simulink model "Final"  (R2022a)
settings: Solver=FixedStepAuto  StartTime=0.0  StopTime=10.0  FixedStep=1e-3  RelTol=1e-3  EnableMultiTasking=on
undefined symbols (not defined in the file): D0, D1, D10, D11, D12, D13, D2, D3, D4, D5, D6, D7, D8, D9, PTA0, PTA1, PTA2, PTB23, PTB9, PTC16, PTC17, PTC2, PTC3, PTC4, PTD0, PTD1, PTD2, PTD3
libraries: frdmk64flib x15
settings Model: ExtModeTrigDuration=5  Creator=pauls  LastModifiedBy=pauls
settings OptimizationCC: EnhancedBackFolding=on  PassReuseOutputArgsAs=Individual arguments  ZeroExternalMemoryAtStartup=off  ZeroInternalMemoryAtStartup=off  MaxStackSize=64  OptimizeBlockOrder=speed  DifferentSizesBufferReuse=on  OptimizationCustomize=off  EfficientTunableParamExpr=on
settings DebuggingCC: ParameterTunabilityLossMsg=error
settings HardwareCC: ProdBitPerPointer=32  ProdBitPerSizeT=32  ProdBitPerPtrDiffT=32  ProdLargestAtomicInteger=Long  ProdLargestAtomicFloat=Double  ProdWordSize=32  ProdHWDeviceType=ARM Compatible->ARM Cortex
settings SFSimCC: MATLABDynamicMemAlloc=off
settings RTWCC: SystemTargetFile=ert.tlc  HardwareBoard=NXP FRDM-K64F  TLCOptions="-aInlineSetEventsForThisBaseRateFcn=TLC_FALSE -aSuppressMultiTaskScheduler=TLC_FALSE  -aRateBasedStepFcn=0"  TemplateMakefile=ert_default_tmf  Toolchain=GNU Tools for ARM Embedded Processors
settings CodeAppCC: ForceParamTrailComments=on  IgnoreCustomStorageClasses=off  OperatorAnnotations=on  SimulinkDataObjDesc=on  SFDataObjDesc=on  InsertBlockDesc=on
settings ERTTargetCC: ExtModeTransport=4  ExtModeMexFile=sendToCommService

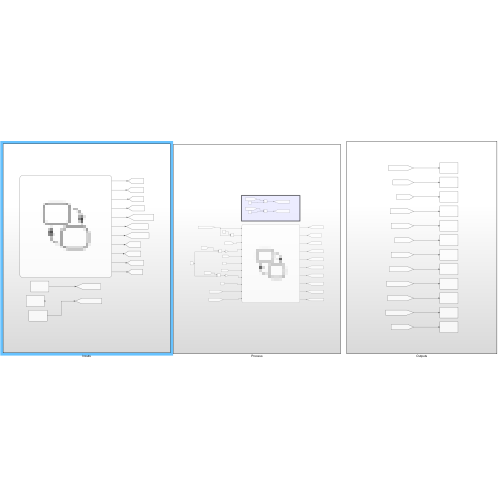
[thumbnail: Simulink's stored preview of the top-level diagram]
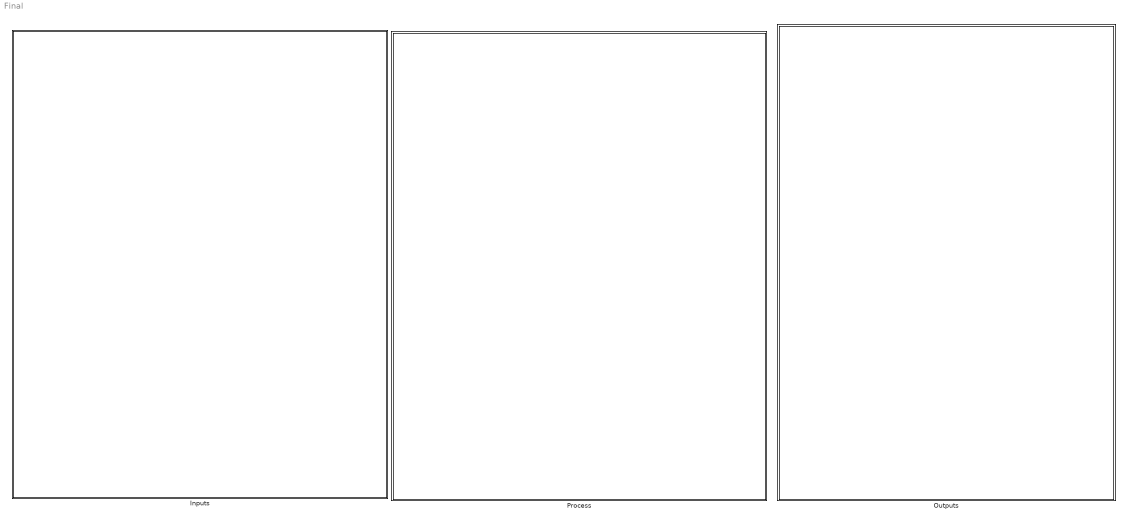
== system Final ==
  Inputs : Subsystem
  Outputs : Subsystem
  Process : Subsystem

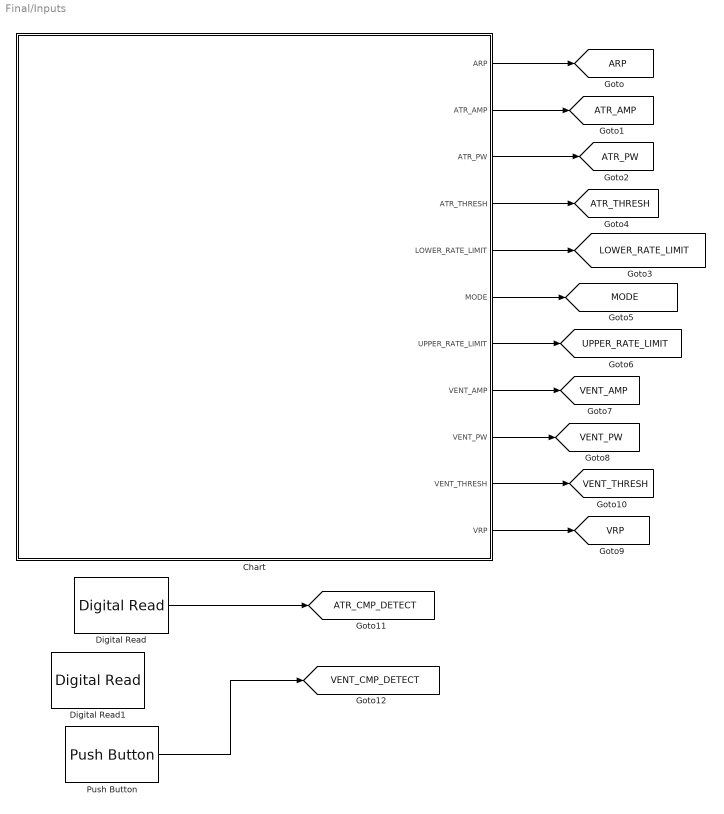
== system Final/Inputs ==
  Chart : Stateflow chart  TreatAsAtomicUnit=on
  Digital Read : frdmk64flib/Digital Read  Whichpin=PTC16 (D0)  SampleTime=-1
  Digital Read1 : frdmk64flib/Digital Read  Whichpin=PTC17 (D1)  SampleTime=-1
  Push Button : frdmk64flib/Push Button  Whichswitch=SW2  SampleTime1=-1
  tag scope: ARP=global, ATR_AMP=global, ATR_CMP_DETECT=global, ATR_PW=global, ATR_THRESH=global, LOWER_RATE_LIMIT=global, MODE=global, UPPER_RATE_LIMIT=global, VENT_AMP=global, VENT_CMP_DETECT=global, VENT_PW=global, VENT_THRESH=global, VRP=global
  wires:
  Chart/1(ARP) -> [ARP]
  Chart/2(ATR_AMP) -> [ATR_AMP]
  Chart/3(ATR_PW) -> [ATR_PW]
  Chart/4(ATR_THRESH) -> [ATR_THRESH]
  Chart/5(LOWER_RATE_LIMIT) -> [LOWER_RATE_LIMIT]
  Chart/6(MODE) -> [MODE]
  Chart/7(UPPER_RATE_LIMIT) -> [UPPER_RATE_LIMIT]
  Chart/8(VENT_AMP) -> [VENT_AMP]
  Chart/9(VENT_PW) -> [VENT_PW]
  Chart/10(VENT_THRESH) -> [VENT_THRESH]
  Chart/11(VRP) -> [VRP]
  Digital Read/1 -> [ATR_CMP_DETECT]
  Push Button/1 -> [VENT_CMP_DETECT]

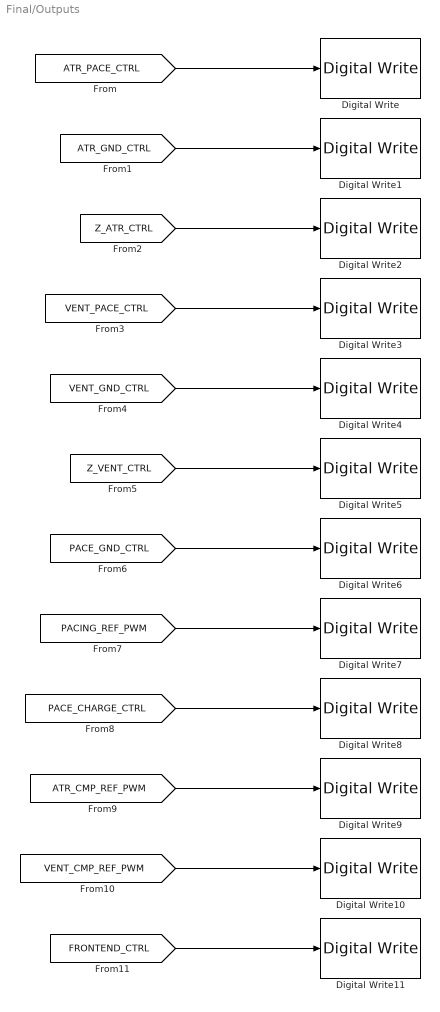
== system Final/Outputs ==
  Digital Write : frdmk64flib/Digital Write  Whichpin=PTA0 (D8)
  Digital Write1 : frdmk64flib/Digital Write  Whichpin=PTD2 (D11)
  Digital Write10 : frdmk64flib/Digital Write  Whichpin=PTA1 (D3)
  Digital Write11 : frdmk64flib/Digital Write  Whichpin=PTD1 (D13)
  Digital Write2 : frdmk64flib/Digital Write  Whichpin=PTB23 (D4)
  Digital Write3 : frdmk64flib/Digital Write  Whichpin=PTC4 (D9)
  Digital Write4 : frdmk64flib/Digital Write  Whichpin=PTD3 (D12)
  Digital Write5 : frdmk64flib/Digital Write  Whichpin=PTC3 (D7)
  Digital Write6 : frdmk64flib/Digital Write  Whichpin=PTD0 (D10)
  Digital Write7 : frdmk64flib/Digital Write  Whichpin=PTA2 (D5)
  Digital Write8 : frdmk64flib/Digital Write  Whichpin=PTB9 (D2)
  Digital Write9 : frdmk64flib/Digital Write  Whichpin=PTC2 (D6)
  wires:
  [ATR_PACE_CTRL] -> Digital Write/1
  [ATR_GND_CTRL] -> Digital Write1/1
  [Z_ATR_CTRL] -> Digital Write2/1
  [VENT_PACE_CTRL] -> Digital Write3/1
  [VENT_GND_CTRL] -> Digital Write4/1
  [PACING_REF_PWM] -> Digital Write7/1
  [Z_VENT_CTRL] -> Digital Write5/1
  [PACE_GND_CTRL] -> Digital Write6/1
  [PACE_CHARGE_CTRL] -> Digital Write8/1
  [FRONTEND_CTRL] -> Digital Write11/1
  [ATR_CMP_REF_PWM] -> Digital Write9/1
  [VENT_CMP_REF_PWM] -> Digital Write10/1

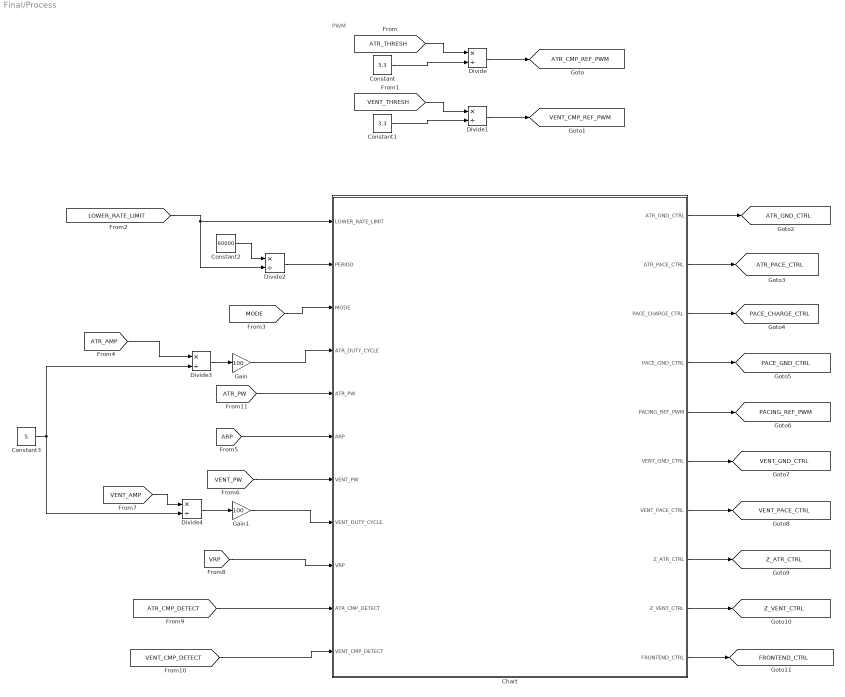
== system Final/Process ==
  note: PWM
  Chart : Stateflow chart  TreatAsAtomicUnit=on
      settings: PortSchema="{\"entries\":[{\"content\":{\"sides\":[{\"content\":{\"connectorIds\":[\"In1\",\"In2\",\"In3\",\"In4\",\"In11\",\"In5\",\"In6\",\"In7\",\"In8\",\"In9\",\"In10\"]},\"type\":\"ConnectorPlacement.EquallySpacedRectSide\",\"uuid\":\"a5edbb4a-33d8-4032-bbc4-520d3a02f21c\"},{\"content\":{\"connectorIds\":[\"Out1\",\"Out2\",\"Out3\",\"Out4\",\"Out5\",\"Out6\",\"Out7\",\"Out8\",\"Out9\",\"Out10\"],\"side\":\"RIGHT\"},\"type\":\"ConnectorPlacement.EquallySpacedRectSide\",\"uuid\":\"7a2184e1-42c4-4433-8732-d8ae781326ee\"},{\"content\":{\"connectorIds\":[],\"side\":\"TOP\"},\"type\":\"ConnectorPlacement.EquallySpacedRectSide\",\"uuid\":\"02a2aeb2-4be5-4b58-8fd3-b17c2c6bfd3f\"}]},\"type\":\"ConnectorPlacement.EquallySpacedConnector\",\"uuid\":\"b8663da6-afa7-4ee6-a0d8-c2d961dca5a7\"}],\"packageUris\":[\"http://schema.mathworks.com/mf0/Connector/R2020b\"],\"version\":\"1.0\"}"
  Constant : Constant  Value=3.3
  Constant1 : Constant  Value=3.3
  Constant2 : Constant  Value=60000
  Constant3 : Constant  Value=5
  Divide{,1..4} (5 alike) : Product  Inputs=*/
  Gain : Gain  Gain=100
  Gain1 : Gain  Gain=100
  tag scope: ATR_CMP_REF_PWM=global, ATR_GND_CTRL=global, ATR_PACE_CTRL=global, FRONTEND_CTRL=global, PACE_CHARGE_CTRL=global, PACE_GND_CTRL=global, PACING_REF_PWM=global, VENT_CMP_REF_PWM=global, VENT_GND_CTRL=global, VENT_PACE_CTRL=global, Z_ATR_CTRL=global, Z_VENT_CTRL=global
  wires:
  [ATR_THRESH] -> Divide/1
  Constant/1 -> Divide/2
  Divide/1 -> [ATR_CMP_REF_PWM]
  Divide1/1 -> [VENT_CMP_REF_PWM]
  Constant1/1 -> Divide1/2
  [VENT_THRESH] -> Divide1/1
  [LOWER_RATE_LIMIT] -> Chart/1(LOWER_RATE_LIMIT), Divide2/2
  Constant2/1 -> Divide2/1
  Divide2/1 -> Chart/2(PERIOD)
  [MODE] -> Chart/3(MODE)
  [ATR_AMP] -> Divide3/1
  Constant3/1 -> Divide3/2, Divide4/2
  Divide3/1 -> Gain/1
  Gain/1 -> Chart/4(ATR_DUTY_CYCLE)
  [ARP] -> Chart/5(ARP)
  [VENT_PW] -> Chart/6(VENT_PW)
  [VENT_AMP] -> Divide4/1
  Divide4/1 -> Gain1/1
  Gain1/1 -> Chart/7(VENT_DUTY_CYCLE)
  [VRP] -> Chart/8(VRP)
  [ATR_CMP_DETECT] -> Chart/9(ATR_CMP_DETECT)
  [VENT_CMP_DETECT] -> Chart/10(VENT_CMP_DETECT)
  [ATR_PW] -> Chart/11(ATR_PW)
  Chart/1(ATR_GND_CTRL) -> [ATR_GND_CTRL]
  Chart/2(ATR_PACE_CTRL) -> [ATR_PACE_CTRL]
  Chart/3(PACE_CHARGE_CTRL) -> [PACE_CHARGE_CTRL]
  Chart/4(PACE_GND_CTRL) -> [PACE_GND_CTRL]
  Chart/5(PACING_REF_PWM) -> [PACING_REF_PWM]
  Chart/6(VENT_GND_CTRL) -> [VENT_GND_CTRL]
  Chart/7(VENT_PACE_CTRL) -> [VENT_PACE_CTRL]
  Chart/8(Z_ATR_CTRL) -> [Z_ATR_CTRL]
  Chart/9(Z_VENT_CTRL) -> [Z_VENT_CTRL]
  Chart/10(FRONTEND_CTRL) -> [FRONTEND_CTRL]

== stateflow chart Final/Inputs/Chart ==
  state Default
    %Setting values to variables
    entry:
    %GENERAL
    MODE = 4 ;%1-AOO, 2- VOO, 3-AAI, 4-VVI
    LOWER_RATE_LIMIT = 60;
    UPPER_RATE_LIMIT = 120;
    %ATRIUM
    ATR_AMP = 3.5;
    ATR_PW = 10;
    ARP = 200;
    ATR_THRESH = 1.8;
    %VENTRICLE
    VENT_AMP = 3.5;
    VENT_PW = 10;
    VRP = 200;
    VENT_THRESH = 2.2;
  (default) -> Default
  data: ARP output; ATR_AMP output; ATR_PW output; ATR_THRESH output; LOWER_RATE_LIMIT output; MODE output; UPPER_RATE_LIMIT output; VENT_AMP output; VENT_PW output; VENT_THRESH output; VRP output

== stateflow chart Final/Process/Chart ==
  state AOO [group]
    state CHARGING
      during:
      %Begin Charging C22 Capacitor
      ATR_PACE_CTRL = LOW
      VENT_PACE_CTRL = LOW
      PACING_REF_PWM = ATR_DUTY_CYCLE
      PACE_CHARGE_CTRL = HIGH
      %Begin Discharging C21 Blocking Capacitor
      PACE_GND_CTRL = HIGH
      VENT_PACE_CTRL = LOW
      Z_ATR_CTRL = LOW
      Z_VENT_CTRL = LOW
      ATR_PACE_CTRL = LOW
      ATR_GND_CTRL = HIGH
      VENT_GND_CTRL = LOW
    state DISCHARGING
      during:
      %Discharge C22 into Atrium (AtrialPacing)
      %Begin Charging C21 Blocking Capacitor
      PACE_CHARGE_CTRL = LOW
      PACE_GND_CTRL = HIGH
      ATR_PACE_CTRL = HIGH
      ATR_GND_CTRL = LOW
      Z_ATR_CTRL = LOW
      Z_VENT_CTRL = LOW
      VENT_GND_CTRL = LOW
      VENT_PACE_CTRL  = LOW
    AOO.CHARGING -> AOO.DISCHARGING [order 1] : after(PERIOD-ATR_PW, msec)
    AOO.DISCHARGING -> AOO.CHARGING : after(ATR_PW, msec)
  state AtStart
  state VOO [group]
    state CHARGING
      during:
      %Begin Charging C22 Capacitor
      ATR_PACE_CTRL = LOW
      VENT_PACE_CTRL = LOW
      PACING_REF_PWM = VENT_DUTY_CYCLE
      PACE_CHARGE_CTRL = HIGH
      %Begin Discharging C21 Blocking Capacitor
      PACE_GND_CTRL = HIGH
      VENT_PACE_CTRL = LOW
      Z_ATR_CTRL = LOW
      Z_VENT_CTRL = LOW
      ATR_PACE_CTRL = LOW
      ATR_GND_CTRL = LOW
      VENT_GND_CTRL = HIGH
    state DISCHARGING
      during:
      %Discharge C22 into Ventricle (Vent Pacing)
      %Begin Charging Blocking Capacitor
      PACE_CHARGE_CTRL = LOW
      PACE_GND_CTRL = HIGH
      ATR_PACE_CTRL = LOW
      ATR_GND_CTRL = LOW
      Z_ATR_CTRL = LOW
      Z_VENT_CTRL = LOW
      VENT_GND_CTRL = LOW
      VENT_PACE_CTRL  = HIGH
    VOO.CHARGING -> VOO.DISCHARGING [order 1] : after(PERIOD-VENT_PW,msec)
    VOO.DISCHARGING -> VOO.CHARGING : after(VENT_PW,msec)
  state AAI [group]
    state PROXY
      during:
      %Discharge C21 Blocking Capacitor
      PACE_GND_CTRL = HIGH
      VENT_PACE_CTRL = LOW
      Z_ATR_CTRL = LOW
      Z_VENT_CTRL = LOW
      ATR_PACE_CTRL = LOW
      ATR_GND_CTRL = HIGH
      VENT_GND_CTRL = LOW
      %Charge C22
      ATR_PACE_CTRL = LOW
      VENT_PACE_CTRL = LOW
      PACING_REF_PWM = ATR_DUTY_CYCLE
      PACE_CHARGE_CTRL = HIGH
    state DISCHARGING
      during:
      %Discharge C22 into Atrium (Atrial Pacing)
      %Begin Charging Blocking Capacitor
      PACE_CHARGE_CTRL = LOW
      PACE_GND_CTRL = HIGH
      ATR_PACE_CTRL = HIGH
      ATR_GND_CTRL = LOW
      Z_ATR_CTRL = LOW
      Z_VENT_CTRL = LOW
      VENT_GND_CTRL = LOW
      VENT_PACE_CTRL  = LOW
    state CHARGING
      during:
      %Begin Charging C22 Capacitor
      ATR_PACE_CTRL = LOW
      VENT_PACE_CTRL = LOW
      PACING_REF_PWM = ATR_DUTY_CYCLE
      PACE_CHARGE_CTRL = HIGH
      %Begin Discharging C21 Blocking Capacitor
      PACE_GND_CTRL = HIGH
      VENT_PACE_CTRL = LOW
      Z_ATR_CTRL = LOW
      Z_VENT_CTRL = LOW
      ATR_PACE_CTRL = LOW
      ATR_GND_CTRL = HIGH
      VENT_GND_CTRL = LOW
    AAI.DISCHARGING -> AAI.PROXY : after(ATR_PW,msec)
    AAI.PROXY -> AAI.CHARGING : after(ARP, msec)
    (junction 12) -> AAI.PROXY : after(LOWER_RATE_LIMIT,msec)
    AAI.CHARGING -> (junction 12) [order 1] : [ATR_CMP_DETECT == HIGH]
    AAI.CHARGING -> AAI.DISCHARGING [order 2] : after(PERIOD-ATR_PW-ARP,msec)
  state VVI [group]
    state PROXY
      during:
      %Step 1
      %Discharge C21 Blocking Capacitor
      PACE_GND_CTRL = HIGH
      VENT_PACE_CTRL = LOW
      Z_ATR_CTRL = LOW
      Z_VENT_CTRL = LOW
      ATR_PACE_CTRL = LOW
      ATR_GND_CTRL = LOW
      VENT_GND_CTRL = HIGH
      %Step 2
      %Charge C22
      ATR_PACE_CTRL = LOW
      VENT_PACE_CTRL = LOW
      PACING_REF_PWM = VENT_DUTY_CYCLE
      PACE_CHARGE_CTRL = HIGH
    state CHARGING
      during:
      %Begin Charging C22 Capacitor
      ATR_PACE_CTRL = LOW
      VENT_PACE_CTRL = LOW
      PACING_REF_PWM = VENT_DUTY_CYCLE
      PACE_CHARGE_CTRL = HIGH
      %Begin Discharging Blocking Capacitor
      PACE_GND_CTRL = HIGH
      VENT_PACE_CTRL = LOW
      Z_ATR_CTRL = LOW
      Z_VENT_CTRL = LOW
      ATR_PACE_CTRL = LOW
      ATR_GND_CTRL = LOW
      VENT_GND_CTRL = HIGH
    state DISCHARGING
      during:
      %Step 1:
      %Discharge C22 into Ventricle (Vent Pacing)
      %Begin Charging Blocking Capacitor
      PACE_CHARGE_CTRL = LOW
      PACE_GND_CTRL = HIGH
      ATR_PACE_CTRL = LOW
      ATR_GND_CTRL = LOW
      Z_ATR_CTRL = LOW
      Z_VENT_CTRL = LOW
      VENT_GND_CTRL = LOW
      VENT_PACE_CTRL  = HIGH
    VVI.DISCHARGING -> VVI.PROXY : after(VENT_PW, msec)
    VVI.PROXY -> VVI.CHARGING : after(VRP, msec)
    (junction 41) -> VVI.PROXY : after(LOWER_RATE_LIMIT,msec)
    VVI.CHARGING -> (junction 41) [order 1] : [VENT_CMP_DETECT ==  HIGH]
    VVI.CHARGING -> VVI.DISCHARGING [order 2] : after(PERIOD-VENT_PW-VRP,msec)
  (default) -> AtStart
  AtStart -> AOO.CHARGING [order 1] : [MODE ==1]
  AtStart -> VVI.CHARGING [order 4] : [MODE == 4]
  AtStart -> AAI.CHARGING [order 3] : [MODE == 3]
  AOO.CHARGING -> AtStart [order 2] : [MODE ~= 1]
  AtStart -> VOO.CHARGING [order 2] : [MODE == 2]
  AAI.CHARGING -> AtStart [order 3] : [MODE ~= 3]
  VVI.CHARGING -> AtStart [order 3] : [MODE ~= 4]
  VOO.CHARGING -> AtStart [order 2] : [MODE ~= 2]
  data: LOWER_RATE_LIMIT input; PERIOD input; MODE input; ATR_DUTY_CYCLE input; ARP input; VENT_PW input; VENT_DUTY_CYCLE input; VRP input; ATR_CMP_DETECT input; VENT_CMP_DETECT input; HIGH local =true; LOW local =false; ATR_GND_CTRL output; ATR_PACE_CTRL output; PACE_CHARGE_CTRL output; PACE_GND_CTRL output; PACING_REF_PWM output; VENT_GND_CTRL output; VENT_PACE_CTRL output; Z_ATR_CTRL output; Z_VENT_CTRL output; ATR_PW input; FRONTEND_CTRL output =true
